simulink library "communications_lib"  (Simulink 8.1)
settings: Solver=ode45  StartTime=0.0  StopTime=10.0  RelTol=1e-3
values from neighbouring files (symbols this model uses):
  Ts = 100E-6    (= 0.0001)    [BANSHEE_init.m]    (also in Ghost_init.m)
libraries: goose_lib x6, rtlab x4, power_quality_lib x4, rtio_generic_modbus x2, DMS_slave_lib x2, LoadProfiles_lib x2, NREL_UDP_lib x2
(part 1 of 2)
settings Model: Creator=re25624  LastModifiedBy=hptb1

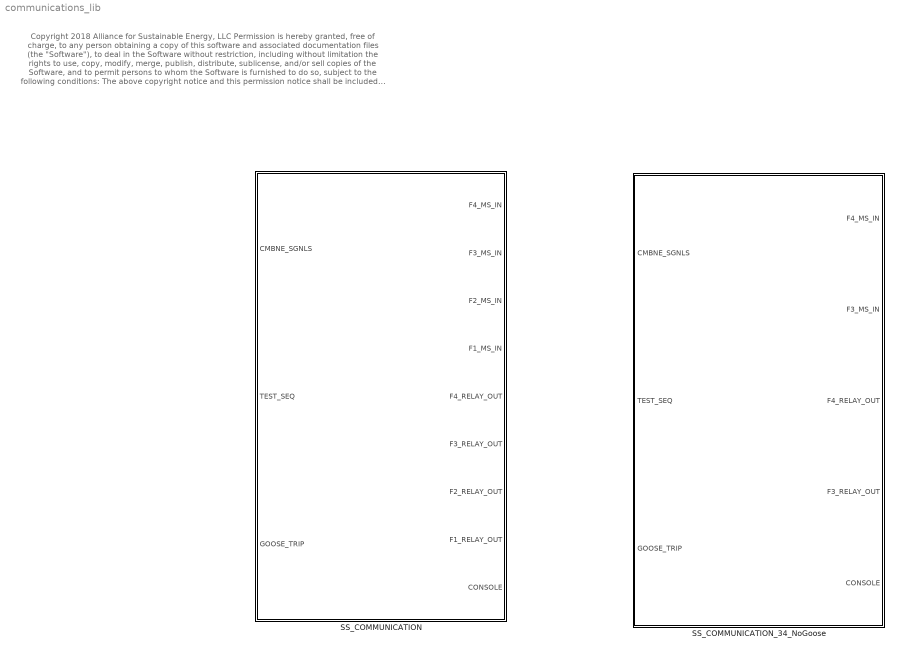
== system communications_lib ==
  note: Copyright 2018 Alliance for Sustainable Energy, LLC
      |
      | Permission is hereby granted, free of charge, to any person obtaining a copy of this software
      | and associated documentation files (the "Software"), to deal in the Software without restriction,
      | including without limitation the rights to use, copy, modify, merge, publish, distribute, sublicense,
      | and/or sell copies of the Software, and to permit persons to whom the Software is furnished to do so,
      | subject to the following conditions:
      |
      | The above copyright notice and this permission notice shall be included in all copies or substantial portions of the Software.
      |
      | THE SOFTWARE IS PROVIDED "AS IS", WITHOUT WARRANTY OF ANY KIND, EXPRESS OR IMPLIED, INCLUDING
      | BUT NOT LIMITED TO THE WARRANTIES OF MERCHANTABILITY, FITNESS FOR A PARTICULAR PURPOSE AND
      | NONINFRINGEMENT. IN NO EVENT SHALL THE AUTHORS, THE COPYRIGHT HOLDERS, THE UNITED STATES,
      | THE UNITED STATES DEPARTMENT OF ENERGY, OR ANY OF THEIR EMPLOYEES BE LIABLE FOR ANY CLAIM,
      | DAMAGES OR OTHER LIABILITY, WHETHER IN AN ACTION OF CONTRACT, TORT OR OTHERWISE, ARISING FROM,
      | OUT OF OR IN CONNECTION WITH THE SOFTWARE OR THE USE OR OTHER DEALINGS IN THE SOFTWARE.
  SS_COMMUNICATION : Subsystem
  SS_COMMUNICATION_34_NoGoose : Subsystem

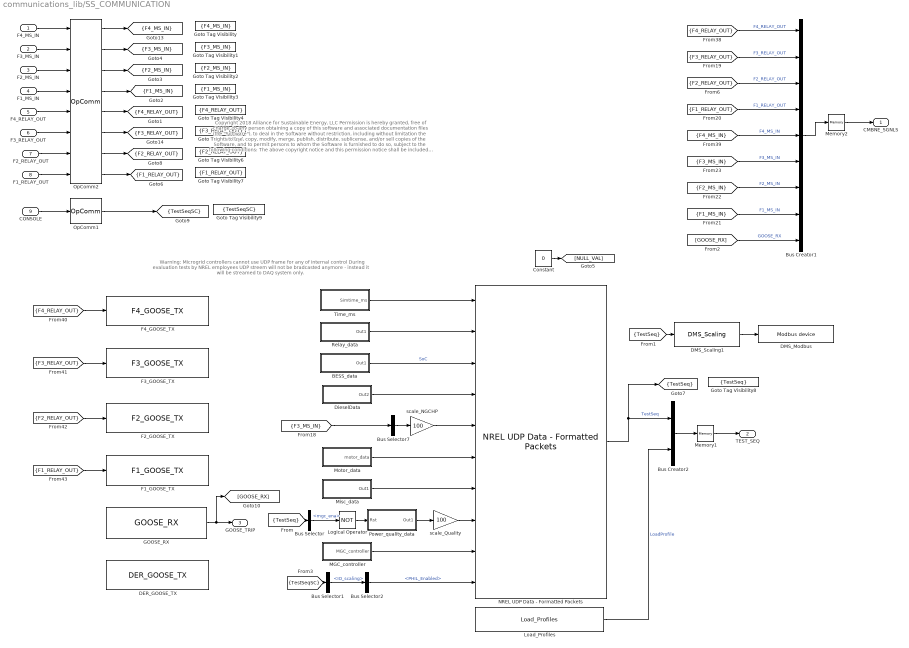
== system communications_lib/SS_COMMUNICATION ==
  note: Copyright 2018 Alliance for Sustainable Energy, LLC
      |
      | Permission is hereby granted, free of charge, to any person obtaining a copy of this software
      | and associated documentation files (the "Software"), to deal in the Software without restriction,
      | including without limitation the rights to use, copy, modify, merge, publish, distribute, sublicense,
      | and/or sell copies of the Software, and to permit persons to whom the Software is furnished to do so,
      | subject to the following conditions:
      |
      | The above copyright notice and this permission notice shall be included in all copies or substantial portions of the Software.
      |
      | THE SOFTWARE IS PROVIDED "AS IS", WITHOUT WARRANTY OF ANY KIND, EXPRESS OR IMPLIED, INCLUDING
      | BUT NOT LIMITED TO THE WARRANTIES OF MERCHANTABILITY, FITNESS FOR A PARTICULAR PURPOSE AND
      | NONINFRINGEMENT. IN NO EVENT SHALL THE AUTHORS, THE COPYRIGHT HOLDERS, THE UNITED STATES,
      | THE UNITED STATES DEPARTMENT OF ENERGY, OR ANY OF THEIR EMPLOYEES BE LIABLE FOR ANY CLAIM,
      | DAMAGES OR OTHER LIABILITY, WHETHER IN AN ACTION OF CONTRACT, TORT OR OTHERWISE, ARISING FROM,
      | OUT OF OR IN CONNECTION WITH THE SOFTWARE OR THE USE OR OTHER DEALINGS IN THE SOFTWARE.
  note: Warning: Microgrid controllers cannot use UDP frame for any of internal control
      | During evaluation tests by NREL employees UDP streem will not be bradcasted anymore - instead it will
      | be streamed to DAQ system only.
  F4_MS_IN : Inport
  F3_MS_IN : Inport  Port=2
  F2_MS_IN : Inport  Port=3
  F1_MS_IN : Inport  Port=4
  F4_RELAY_OUT : Inport  Port=5
  F3_RELAY_OUT : Inport  Port=6
  F2_RELAY_OUT : Inport  Port=7
  F1_RELAY_OUT : Inport  Port=8
  CONSOLE : Inport  Port=9
  BESS_data : Subsystem
  Bus Creator1 : BusCreator  Inputs=9
  Bus Creator2 : BusCreator  Inputs=2
  Bus Selector : BusSelector  OutputSignals=misc.mgc_ena
  Bus Selector1 : BusSelector  OutputSignals=IO_scaling
  Bus Selector2 : BusSelector  OutputSignals=PHIL_Enabled
  Bus Selector7 : BusSelector  OutputSignals=NG_CHP_DATA.cb.relay_out.m.Vpu,NG_CHP_DATA.CHPData.TempActual,NG_CHP_DATA.CHPData.Thermal data.Heat_Recovered_MBtu_hr,NG_CHP_DATA.CHPData.Thermal data.Nm3_per_hour_NG_fuel_usage,NG_CHP_DATA.CHPData.Thermal data.CO2_lbm_hr,NG_CHP_DATA.CHPData.HeatFromBoiler MBtu/hr,NG_CHP_DATA.CHPData.CHPHeatContribution MBtu/hr,NG_CHP_DATA.CHPData.Boiler_Nm^3/hr ,NG_CHP_DATA.CHPData.Boiler lbm/hr CO2  OutputAsBus=on
  Constant : Constant  Value=0
  DER_GOOSE_TX : goose_lib/DER_GOOSE_TX
  DMS_Modbus : rtio_generic_modbus/Modbus device  conf_name=DMS_cfg.opal  conf_name_mask=DMS_cfg.xls  sample_time=Ts
  DMS_Scaling1 : DMS_slave_lib/DMS_Scaling
  DieselData : Subsystem
  F1_GOOSE_TX : goose_lib/F1_GOOSE_TX
  F2_GOOSE_TX : goose_lib/F2_GOOSE_TX
  F3_GOOSE_TX : goose_lib/F3_GOOSE_TX
  F4_GOOSE_TX : goose_lib/F4_GOOSE_TX
  "GOOSE_RX " : goose_lib/GOOSE_RX 
  Goto Tag Visibility : GotoTagVisibility  GotoTag=F4_MS_IN
  Goto Tag Visibility1 : GotoTagVisibility  GotoTag=F3_MS_IN
  Goto Tag Visibility2 : GotoTagVisibility  GotoTag=F2_MS_IN
  Goto Tag Visibility3 : GotoTagVisibility  GotoTag=F1_MS_IN
  Goto Tag Visibility4 : GotoTagVisibility  GotoTag=F4_RELAY_OUT
  Goto Tag Visibility5 : GotoTagVisibility  GotoTag=F3_RELAY_OUT
  Goto Tag Visibility6 : GotoTagVisibility  GotoTag=F2_RELAY_OUT
  Goto Tag Visibility7 : GotoTagVisibility  GotoTag=F1_RELAY_OUT
  Goto Tag Visibility8 : GotoTagVisibility  GotoTag=TestSeq
  Goto Tag Visibility9 : GotoTagVisibility  GotoTag=TestSeqSC
  Load_Profiles : LoadProfiles_lib/Load_Profiles
  Logical Operator : Logic  Operator=NOT  AllPortsSameDT=off  OutDataTypeStr=boolean
  MGC_controller : Subsystem
  Memory1 : Memory
  Memory2 : Memory
  Misc_data : Subsystem
  Motor_data : Subsystem
  NREL UDP Data - Formatted Packets : NREL_UDP_lib/NREL UDP Data - Formatted Packets  ProfileID=6  NumOfRelays=[59, [1, 1, 1000, 100]]  NumOfBatteries=2  NumOfDieselGensets=[2, [100, 100]]  NumOfNGCHPGensets=[1, [100, 100, 100, 100, 100, 100, 100, 100, 100]]  NumOfMotors=2  NumOfQuality=[23 10 10]  NumOfMiscellaneousDataScales=2  NumOfMiscellaneousDataSignalsScales=[[50, 1], [8, 1]]
  OpComm1 : rtlab/OpComm  nbport=1  groupe_acq=1  subsys_rate=0  st=0  Synchronization=on  Interpolation=on  Threshold=1.0  Missed_Data=off  Sim_Time=off  Samples=off  dynSigOut=off  from_console=1  warning_done=off  writeOpCommFile=off  Offset=off
  OpComm2 : rtlab/OpComm  nbport=8  groupe_acq=1  subsys_rate=0  st=0  Synchronization=on  Interpolation=on  Threshold=1.0  Missed_Data=off  Sim_Time=off  Samples=off  dynSigOut=off  from_console=0  warning_done=off  writeOpCommFile=off  Offset=off
  Power_quality_data : Subsystem
  Relay_data : Subsystem
  Time_ms : Subsystem
  scale_NGCHP : Gain  Gain=100
  scale_Quality : Gain  Gain=100
  CMBNE_SGNLS : Outport
  TEST_SEQ : Outport  Port=2
  GOOSE_TRIP : Outport  Port=3
  tag scope: F1_MS_IN=scoped, F1_RELAY_OUT=scoped, F2_MS_IN=scoped, F2_RELAY_OUT=scoped, F3_MS_IN=scoped, F3_RELAY_OUT=scoped, F4_MS_IN=scoped, F4_RELAY_OUT=scoped, TestSeq=scoped, TestSeqSC=scoped
  wires:
  Bus Selector2/1 -> NREL UDP Data - Formatted Packets/10  "<PHIL_Enabled>"
  Bus Selector1/1 -> Bus Selector2/1  "<IO_scaling>"
  [TestSeqSC] -> Bus Selector1/1
  [GOOSE_RX] -> Bus Creator1/9  "GOOSE_RX"
  MGC_controller/1(MGC_controller) -> NREL UDP Data - Formatted Packets/9
  DMS_Scaling1/1 -> DMS_Modbus/1
  [TestSeq] -> DMS_Scaling1/1
  scale_Quality/1 -> NREL UDP Data - Formatted Packets/8
  Logical Operator/1 -> Power_quality_data/1(Rst)
  Bus Selector/1 -> Logical Operator/1  "<mgc_ena>"
  [TestSeq] -> Bus Selector/1
  Power_quality_data/1(Out1) -> scale_Quality/1
  DieselData/1(Out2) -> NREL UDP Data - Formatted Packets/4
  BESS_data/1(Out1) -> NREL UDP Data - Formatted Packets/3  "SoC"
  OpComm1/1 -> [TestSeqSC]
  CONSOLE/1 -> OpComm1/1
  Bus Creator2/1 -> Memory1/1
  NREL UDP Data - Formatted Packets/1 -> Bus Creator2/1, [TestSeq]  "TestSeq"
  Motor_data/1(motor_data) -> NREL UDP Data - Formatted Packets/6
  Misc_data/1(Out1) -> NREL UDP Data - Formatted Packets/7
  Relay_data/1(Out1) -> NREL UDP Data - Formatted Packets/2
  "GOOSE_RX "/1 -> GOOSE_TRIP/1, [GOOSE_RX]
  [F1_RELAY_OUT] -> F1_GOOSE_TX/1
  [F2_RELAY_OUT] -> F2_GOOSE_TX/1
  [F3_RELAY_OUT] -> F3_GOOSE_TX/1
  [F4_RELAY_OUT] -> F4_GOOSE_TX/1
  [F4_MS_IN] -> Bus Creator1/5  "F4_MS_IN"
  [F4_RELAY_OUT] -> Bus Creator1/1  "F4_RELAY_OUT"
  OpComm2/8 -> [F1_RELAY_OUT]
  OpComm2/7 -> [F2_RELAY_OUT]
  OpComm2/6 -> [F3_RELAY_OUT]
  OpComm2/5 -> [F4_RELAY_OUT]
  OpComm2/4 -> [F1_MS_IN]
  OpComm2/3 -> [F2_MS_IN]
  OpComm2/2 -> [F3_MS_IN]
  OpComm2/1 -> [F4_MS_IN]
  F3_RELAY_OUT/1 -> OpComm2/6
  F4_RELAY_OUT/1 -> OpComm2/5
  F4_MS_IN/1 -> OpComm2/1
  Time_ms/1(Simtime_ms) -> NREL UDP Data - Formatted Packets/1
  [F2_MS_IN] -> Bus Creator1/7  "F2_MS_IN"
  [F3_MS_IN] -> Bus Creator1/6  "F3_MS_IN"
  [F3_RELAY_OUT] -> Bus Creator1/2  "F3_RELAY_OUT"
  [F1_RELAY_OUT] -> Bus Creator1/4  "F1_RELAY_OUT"
  [F2_RELAY_OUT] -> Bus Creator1/3  "F2_RELAY_OUT"
  [F1_MS_IN] -> Bus Creator1/8  "F1_MS_IN"
  Bus Creator1/1 -> Memory2/1
  Memory2/1 -> CMBNE_SGNLS/1
  scale_NGCHP/1 -> NREL UDP Data - Formatted Packets/5
  Bus Selector7/1 -> scale_NGCHP/1
  [F3_MS_IN] -> Bus Selector7/1
  Constant/1 -> [NULL_VAL]
  F1_MS_IN/1 -> OpComm2/4
  F2_MS_IN/1 -> OpComm2/3
  F1_RELAY_OUT/1 -> OpComm2/8
  F2_RELAY_OUT/1 -> OpComm2/7
  Memory1/1 -> TEST_SEQ/1
  F3_MS_IN/1 -> OpComm2/2
  Load_Profiles/1 -> Bus Creator2/2  "LoadProfile"

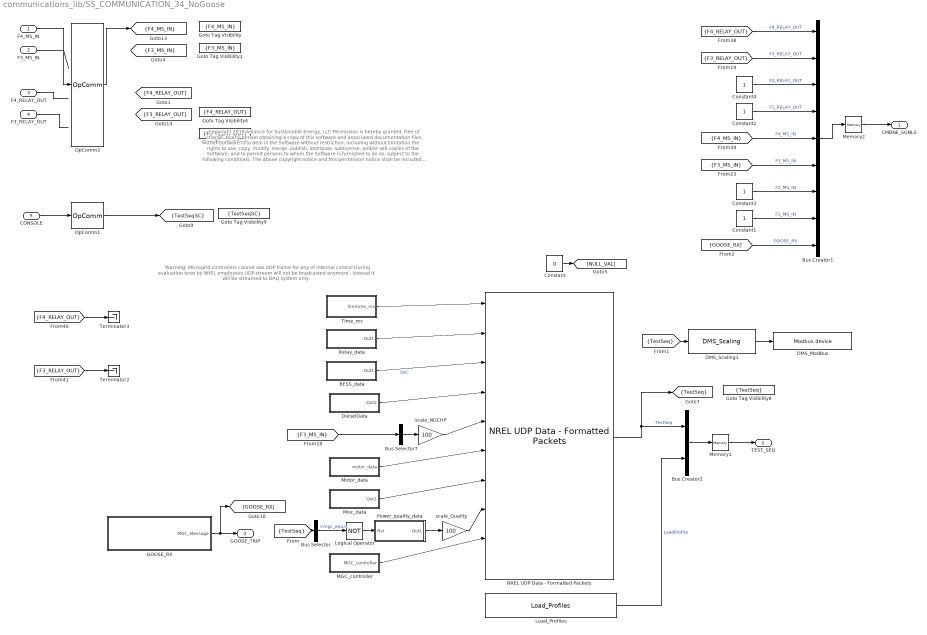
== system communications_lib/SS_COMMUNICATION_34_NoGoose ==
  note: Warning: Microgrid controllers cannot use UDP frame for any of internal control
      | During evaluation tests by NREL employees UDP streem will not be bradcasted anymore - instead it will
      | be streamed to DAQ system only.
  note: Copyright 2018 Alliance for Sustainable Energy, LLC
      |
      | Permission is hereby granted, free of charge, to any person obtaining a copy of this software
      | and associated documentation files (the "Software"), to deal in the Software without restriction,
      | including without limitation the rights to use, copy, modify, merge, publish, distribute, sublicense,
      | and/or sell copies of the Software, and to permit persons to whom the Software is furnished to do so,
      | subject to the following conditions:
      |
      | The above copyright notice and this permission notice shall be included in all copies or substantial portions of the Software.
      |
      | THE SOFTWARE IS PROVIDED "AS IS", WITHOUT WARRANTY OF ANY KIND, EXPRESS OR IMPLIED, INCLUDING
      | BUT NOT LIMITED TO THE WARRANTIES OF MERCHANTABILITY, FITNESS FOR A PARTICULAR PURPOSE AND
      | NONINFRINGEMENT. IN NO EVENT SHALL THE AUTHORS, THE COPYRIGHT HOLDERS, THE UNITED STATES,
      | THE UNITED STATES DEPARTMENT OF ENERGY, OR ANY OF THEIR EMPLOYEES BE LIABLE FOR ANY CLAIM,
      | DAMAGES OR OTHER LIABILITY, WHETHER IN AN ACTION OF CONTRACT, TORT OR OTHERWISE, ARISING FROM,
      | OUT OF OR IN CONNECTION WITH THE SOFTWARE OR THE USE OR OTHER DEALINGS IN THE SOFTWARE.
  F4_MS_IN : Inport
  F3_MS_IN : Inport  Port=2
  F4_RELAY_OUT : Inport  Port=3
  F3_RELAY_OUT : Inport  Port=4
  CONSOLE : Inport  Port=5
  BESS_data : Subsystem
  Bus Creator1 : BusCreator  Inputs=9
  Bus Creator2 : BusCreator  Inputs=2
  Bus Selector : BusSelector  OutputSignals=misc.mgc_ena
  Bus Selector7 : BusSelector  OutputSignals=NG_CHP_DATA.cb.relay_out.m.Vpu,NG_CHP_DATA.CHPData.TempActual,NG_CHP_DATA.CHPData.Thermal data.Heat_Recovered_MBtu_hr,NG_CHP_DATA.CHPData.Thermal data.Nm3_per_hour_NG_fuel_usage,NG_CHP_DATA.CHPData.Thermal data.CO2_lbm_hr,NG_CHP_DATA.CHPData.HeatFromBoiler MBtu/hr,NG_CHP_DATA.CHPData.CHPHeatContribution MBtu/hr,NG_CHP_DATA.CHPData.Boiler_Nm^3/hr ,NG_CHP_DATA.CHPData.Boiler lbm/hr CO2  OutputAsBus=on
  Constant : Constant  Value=0
  Constant{1..4} (4 alike) : Constant
  DMS_Modbus : rtio_generic_modbus/Modbus device  conf_name=DMS_cfg.opal  conf_name_mask=DMS_cfg.xls  sample_time=Ts
  DMS_Scaling1 : DMS_slave_lib/DMS_Scaling
  DieselData : Subsystem
  "GOOSE_RX " : Subsystem
  Goto Tag Visibility : GotoTagVisibility  GotoTag=F4_MS_IN
  Goto Tag Visibility1 : GotoTagVisibility  GotoTag=F3_MS_IN
  Goto Tag Visibility4 : GotoTagVisibility  GotoTag=F4_RELAY_OUT
  Goto Tag Visibility5 : GotoTagVisibility  GotoTag=F3_RELAY_OUT
  Goto Tag Visibility8 : GotoTagVisibility  GotoTag=TestSeq
  Goto Tag Visibility9 : GotoTagVisibility  GotoTag=TestSeqSC
  Load_Profiles : LoadProfiles_lib/Load_Profiles
  Logical Operator : Logic  Operator=NOT  AllPortsSameDT=off  OutDataTypeStr=boolean
  MGC_controller : Subsystem
  Memory1 : Memory
  Memory2 : Memory
  Misc_data : Subsystem
  Motor_data : Subsystem
  NREL UDP Data - Formatted Packets : NREL_UDP_lib/NREL UDP Data - Formatted Packets  ProfileID=6  NumOfRelays=[59, [1, 1, 1000, 100]]  NumOfBatteries=2  NumOfDieselGensets=[2, [100, 100]]  NumOfNGCHPGensets=[1, [100, 100, 100, 100, 100, 100, 100, 100, 100]]  NumOfMotors=2  NumOfQuality=[23 10 10]  NumOfMiscellaneousDataScales=2  NumOfMiscellaneousDataSignalsScales=[[50, 1], [8, 1]]
  OpComm1 : rtlab/OpComm  nbport=1  groupe_acq=1  subsys_rate=0  st=0  Synchronization=on  Interpolation=on  Threshold=1.0  Missed_Data=off  Sim_Time=off  Samples=off  dynSigOut=off  from_console=1  warning_done=off  writeOpCommFile=off  Offset=off
  OpComm2 : rtlab/OpComm  nbport=4  groupe_acq=1  subsys_rate=0  st=0  Synchronization=on  Interpolation=on  Threshold=1.0  Missed_Data=off  Sim_Time=off  Samples=off  dynSigOut=off  from_console=0  warning_done=off  writeOpCommFile=off  Offset=off
  Power_quality_data : Subsystem
  Relay_data : Subsystem
  Terminator2 : Terminator
  Terminator3 : Terminator
  Time_ms : Subsystem
  scale_NGCHP : Gain  Gain=100
  scale_Quality : Gain  Gain=100
  CMBNE_SGNLS : Outport
  TEST_SEQ : Outport  Port=2
  GOOSE_TRIP : Outport  Port=3
  tag scope: F3_MS_IN=scoped, F3_RELAY_OUT=scoped, F4_MS_IN=scoped, F4_RELAY_OUT=scoped, TestSeq=scoped, TestSeqSC=scoped
  wires:
  [GOOSE_RX] -> Bus Creator1/9  "GOOSE_RX"
  MGC_controller/1(MGC_controller) -> NREL UDP Data - Formatted Packets/9
  DMS_Scaling1/1 -> DMS_Modbus/1
  [TestSeq] -> DMS_Scaling1/1
  scale_Quality/1 -> NREL UDP Data - Formatted Packets/8
  Logical Operator/1 -> Power_quality_data/1(Rst)
  Bus Selector/1 -> Logical Operator/1  "<mgc_ena>"
  [TestSeq] -> Bus Selector/1
  Power_quality_data/1(Out1) -> scale_Quality/1
  DieselData/1(Out2) -> NREL UDP Data - Formatted Packets/4
  BESS_data/1(Out1) -> NREL UDP Data - Formatted Packets/3  "SoC"
  OpComm1/1 -> [TestSeqSC]
  CONSOLE/1 -> OpComm1/1
  Bus Creator2/1 -> Memory1/1
  NREL UDP Data - Formatted Packets/1 -> Bus Creator2/1, [TestSeq]  "TestSeq"
  Motor_data/1(motor_data) -> NREL UDP Data - Formatted Packets/6
  Misc_data/1(Out1) -> NREL UDP Data - Formatted Packets/7
  Relay_data/1(Out1) -> NREL UDP Data - Formatted Packets/2
  "GOOSE_RX "/1(MGC_Message) -> GOOSE_TRIP/1, [GOOSE_RX]
  [F3_RELAY_OUT] -> Terminator2/1
  [F4_RELAY_OUT] -> Terminator3/1
  [F4_MS_IN] -> Bus Creator1/5  "F4_MS_IN"
  [F4_RELAY_OUT] -> Bus Creator1/1  "F4_RELAY_OUT"
  ? -> [F3_RELAY_OUT]
  ? -> [F4_RELAY_OUT]
  ? -> [F3_MS_IN]
  OpComm2/1 -> [F4_MS_IN]
  F3_RELAY_OUT/1 -> ?
  F4_RELAY_OUT/1 -> ?
  F4_MS_IN/1 -> OpComm2/1
  Time_ms/1(Simtime_ms) -> NREL UDP Data - Formatted Packets/1
  Constant3/1 -> Bus Creator1/7  "F2_MS_IN"
  [F3_MS_IN] -> Bus Creator1/6  "F3_MS_IN"
  [F3_RELAY_OUT] -> Bus Creator1/2  "F3_RELAY_OUT"
  Constant2/1 -> Bus Creator1/4  "F1_RELAY_OUT"
  Constant4/1 -> Bus Creator1/3  "F2_RELAY_OUT"
  Constant1/1 -> Bus Creator1/8  "F1_MS_IN"
  Bus Creator1/1 -> Memory2/1
  Memory2/1 -> CMBNE_SGNLS/1
  scale_NGCHP/1 -> NREL UDP Data - Formatted Packets/5
  Bus Selector7/1 -> scale_NGCHP/1
  [F3_MS_IN] -> Bus Selector7/1
  Constant/1 -> [NULL_VAL]
  Memory1/1 -> TEST_SEQ/1
  F3_MS_IN/1 -> ?
  Load_Profiles/1 -> Bus Creator2/2  "LoadProfile"

== system communications_lib/SS_COMMUNICATION/BESS_data ==
  note: 0 .... 10000
      | 0 ... 100%
  Bus Selector1 : BusSelector  OutputSignals=Battery.SoC
  Bus Selector2 : BusSelector  OutputSignals=Battery.SoC
  Bus Selector3 : BusSelector  OutputSignals=ESS_DATA
  Bus Selector9 : BusSelector  OutputSignals=ESS_DATA
  Mux : Mux  Inputs=2
  Scale_SoC : Gain  Gain=100
  Out1 : Outport
  wires:
  [F2_MS_IN] -> Bus Selector3/1
  Bus Selector3/1 -> Bus Selector2/1  "<ESS_DATA>"
  Bus Selector2/1 -> Mux/1  "<SoC>"
  Scale_SoC/1 -> Out1/1
  [F4_MS_IN] -> Bus Selector9/1
  Bus Selector9/1 -> Bus Selector1/1  "<ESS_DATA>"
  Bus Selector1/1 -> Mux/2  "<SoC>"
  Mux/1 -> Scale_SoC/1

== system communications_lib/SS_COMMUNICATION/DieselData ==
  Bus Selector : BusSelector  OutputSignals=GEN3_DATA.gen.gal_per_hr,GEN3_DATA.cb.relay_out.m.Vpu
  Bus Selector1 : BusSelector  OutputSignals=DIESEL_DATA.gen.gal_per_hr,DIESEL_DATA.cb.relay_out.m.Vpu
  Mux : Mux
  scale_diesel3 : Gain  Gain=100
  Out2 : Outport
  wires:
  Bus Selector1/2 -> Mux/3  "<Vpu>"
  scale_diesel3/1 -> Out2/1
  [F1_MS_IN] -> Bus Selector1/1
  [F4_MS_IN] -> Bus Selector/1
  Bus Selector/1 -> Mux/2  "<gal_per_hr>"
  Bus Selector1/1 -> Mux/1  "<gal_per_hr>"
  Mux/1 -> scale_diesel3/1
  Bus Selector/2 -> Mux/4  "<Vpu>"

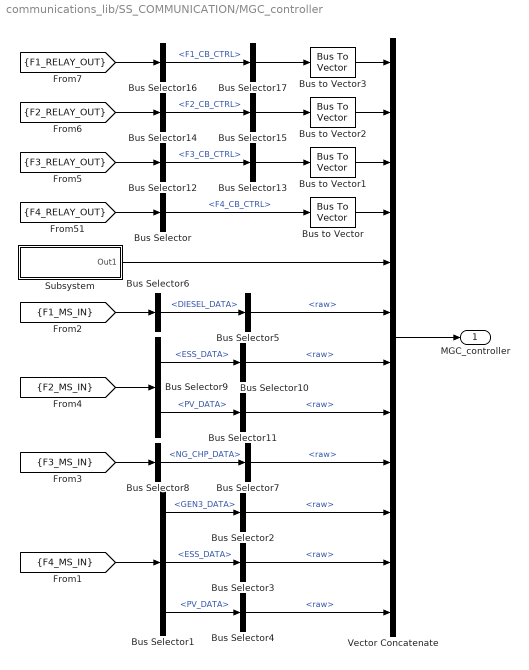
== system communications_lib/SS_COMMUNICATION/MGC_controller ==
  Bus Selector : BusSelector  OutputSignals=F4_CB_CTRL
  Bus Selector1 : BusSelector  OutputSignals=GEN3_DATA,ESS_DATA,PV_DATA
  Bus Selector{3..4,10..11} (4 alike) : BusSelector  OutputSignals=raw
  Bus Selector12 : BusSelector  OutputSignals=F3_CB_CTRL
  Bus Selector13 : BusSelector  OutputSignals=signal1,signal2,signal3,signal4,signal5,signal6,signal7,signal8,signal9,signal10  OutputAsBus=on
  Bus Selector14 : BusSelector  OutputSignals=F2_CB_CTRL
  Bus Selector15 : BusSelector  OutputSignals=signal1,signal2,signal3,signal4,signal5,signal6,signal7,signal8,signal9,signal10,signal11,signal12,signal13,signal14,signal15,signal16,signal17,signal18,signal19  OutputAsBus=on
  Bus Selector16 : BusSelector  OutputSignals=F1_CB_CTRL
  Bus Selector17 : BusSelector  OutputSignals=signal1,signal2,signal3,signal4,signal5,signal6,signal7,signal8,signal9,signal10,signal11,signal12,signal13,signal14  OutputAsBus=on
  Bus Selector2 : BusSelector  OutputSignals=ctrl.raw
  Bus Selector5 : BusSelector  OutputSignals=ctrl.raw
  Bus Selector6 : BusSelector  OutputSignals=DIESEL_DATA
  Bus Selector7 : BusSelector  OutputSignals=ctrl.raw
  Bus Selector8 : BusSelector  OutputSignals=NG_CHP_DATA
  Bus Selector9 : BusSelector  OutputSignals=ESS_DATA,PV_DATA
  Bus to Vector{,1..3} (4 alike) : BusToVector
  Subsystem : Subsystem
      mask Display: disp('PCC control');
  Vector Concatenate : Concatenate  NumInputs=12
  MGC_controller : Outport
  wires:
  Bus Selector17/1 -> Bus to Vector3/1
  Bus Selector16/1 -> Bus Selector17/1  "<F1_CB_CTRL>"
  [F1_RELAY_OUT] -> Bus Selector16/1
  Bus to Vector3/1 -> Vector Concatenate/1
  Bus Selector15/1 -> Bus to Vector2/1
  Bus Selector14/1 -> Bus Selector15/1  "<F2_CB_CTRL>"
  [F2_RELAY_OUT] -> Bus Selector14/1
  Bus to Vector2/1 -> Vector Concatenate/2
  Bus Selector13/1 -> Bus to Vector1/1
  Bus Selector12/1 -> Bus Selector13/1  "<F3_CB_CTRL>"
  [F3_RELAY_OUT] -> Bus Selector12/1
  Bus to Vector/1 -> Vector Concatenate/4
  Bus Selector9/2 -> Bus Selector11/1  "<PV_DATA>"
  Bus Selector9/1 -> Bus Selector10/1  "<ESS_DATA>"
  Bus Selector11/1 -> Vector Concatenate/8  "<raw>"
  Bus Selector10/1 -> Vector Concatenate/7  "<raw>"
  [F2_MS_IN] -> Bus Selector9/1
  Bus Selector4/1 -> Vector Concatenate/12  "<raw>"
  Bus Selector8/1 -> Bus Selector7/1  "<NG_CHP_DATA>"
  [F3_MS_IN] -> Bus Selector8/1
  Bus Selector7/1 -> Vector Concatenate/9  "<raw>"
  Bus Selector6/1 -> Bus Selector5/1  "<DIESEL_DATA>"
  [F1_MS_IN] -> Bus Selector6/1
  Vector Concatenate/1 -> MGC_controller/1
  Subsystem/1(Out1) -> Vector Concatenate/5
  Bus to Vector1/1 -> Vector Concatenate/3
  Bus Selector/1 -> Bus to Vector/1  "<F4_CB_CTRL>"
  [F4_RELAY_OUT] -> Bus Selector/1
  [F4_MS_IN] -> Bus Selector1/1
  Bus Selector1/1 -> Bus Selector2/1  "<GEN3_DATA>"
  Bus Selector1/2 -> Bus Selector3/1  "<ESS_DATA>"
  Bus Selector1/3 -> Bus Selector4/1  "<PV_DATA>"
  Bus Selector3/1 -> Vector Concatenate/11  "<raw>"
  Bus Selector2/1 -> Vector Concatenate/10  "<raw>"
  Bus Selector5/1 -> Vector Concatenate/6  "<raw>"

== system communications_lib/SS_COMMUNICATION/Misc_data ==
  note: Data ordered as:
      | I-P-C
      | kW-VRMSLL
  Bus Creator : BusCreator
  Constant : Constant  Value=zeros(1,9)
  Mux8 : Mux  Inputs=2
  Mux9 : Mux  Inputs=2
  Subsystem : Subsystem
  Subsystem1 : Subsystem
  scale_load : Gain
  Out1 : Outport
  wires:
  Subsystem1/1(Out1) -> Mux8/2
  Subsystem/1(Out1) -> Mux8/1
  [F4_MS_IN] -> Bus Creator/1  "F4"
  Mux9/1 -> Out1/1
  Constant/1 -> Mux9/2
  Mux8/1 -> scale_load/1
  Bus Creator/1 -> Subsystem/1(In1), Subsystem1/1(In1)
  [F1_MS_IN] -> Bus Creator/4  "F1"
  [F2_MS_IN] -> Bus Creator/3  "F2"
  [F3_MS_IN] -> Bus Creator/2  "F3"
  scale_load/1 -> Mux9/1

== system communications_lib/SS_COMMUNICATION/Motor_data ==
  note: kW
      | kVAR
      | VLL_RMS
      | RPM
  Bus Selector1 : BusSelector  OutputSignals=MOTOR_DATA
  Bus Selector2 : BusSelector  OutputSignals=kW,kVAr,VRMSLL,RPM  OutputAsBus=on
  Bus Selector3 : BusSelector  OutputSignals=MOTOR_DATA
  Bus Selector4 : BusSelector  OutputSignals=kW,kVAr,VRMSLL,RPM  OutputAsBus=on
  Bus to Vector : BusToVector
  Bus to Vector1 : BusToVector
  Mux5 : Mux  Inputs=2
  motor_data : Outport
  wires:
  Bus Selector4/1 -> Bus to Vector1/1
  Bus Selector3/1 -> Bus Selector4/1  "<MOTOR_DATA>"
  [F3_MS_IN] -> Bus Selector3/1
  Bus to Vector1/1 -> Mux5/2  "Motor2"
  Bus Selector2/1 -> Bus to Vector/1
  Bus Selector1/1 -> Bus Selector2/1  "<MOTOR_DATA>"
  [F1_MS_IN] -> Bus Selector1/1
  Bus to Vector/1 -> Mux5/1  "Motor1"
  Mux5/1 -> motor_data/1

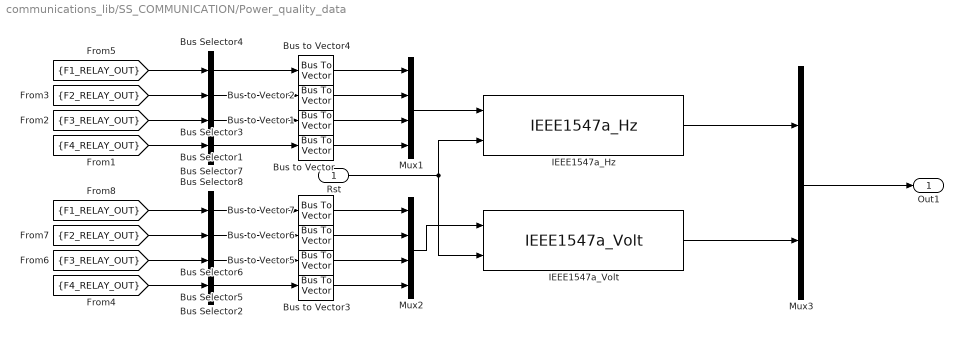
== system communications_lib/SS_COMMUNICATION/Power_quality_data ==
  Rst : Inport
  Bus Selector1 : BusSelector  OutputSignals=F3_CB_1.m.Hz,F3_CB_5.m.Hz,F3_CB_7.m.Hz,F3_CB_8.m.Hz,F3_CB_9.m.Hz  OutputAsBus=on
  Bus Selector2 : BusSelector  OutputSignals=F4_CB_1.m.Vpu,F4_CB_2.m.Vpu,F4_CB_5.m.Vpu  OutputAsBus=on
  Bus Selector3 : BusSelector  OutputSignals=F2_CB_1.m.Hz,F2_CB_6.m.Hz,F2_CB_8.m.Hz,F2_CB_9.m.Hz,F2_CB_12.m.Hz,F2_CB_14.m.Hz,F2_CB_16.m.Hz,F2_CB_17.m.Hz,F2_CB_19.m.Hz  OutputAsBus=on
  Bus Selector4 : BusSelector  OutputSignals=F1_CB_1.m.Hz,F1_CB_4.m.Hz,F1_CB_9.m.Hz,F1_CB_6.m.Hz,F1_CB_10.m.Hz,F1_CB_14.m.Hz  OutputAsBus=on
  Bus Selector5 : BusSelector  OutputSignals=F3_CB_1.m.Vpu,F3_CB_5.m.Vpu,F3_CB_7.m.Vpu,F3_CB_8.m.Vpu,F3_CB_9.m.Vpu  OutputAsBus=on
  Bus Selector6 : BusSelector  OutputSignals=F2_CB_1.m.Vpu,F2_CB_6.m.Vpu,F2_CB_8.m.Vpu,F2_CB_9.m.Vpu,F2_CB_12.m.Vpu,F2_CB_14.m.Vpu,F2_CB_16.m.Vpu,F2_CB_17.m.Vpu,F2_CB_19.m.Vpu  OutputAsBus=on
  Bus Selector7 : BusSelector  OutputSignals=F4_CB_1.m.Hz,F4_CB_2.m.Hz,F4_CB_5.m.Hz  OutputAsBus=on
  Bus Selector8 : BusSelector  OutputSignals=F1_CB_1.m.Vpu,F1_CB_4.m.Vpu,F1_CB_9.m.Vpu,F1_CB_6.m.Vpu,F1_CB_10.m.Vpu,F1_CB_14.m.Vpu  OutputAsBus=on
  Bus to Vector{,1..7} (8 alike) : BusToVector
  IEEE1547a_Hz : power_quality_lib/IEEE1547a_Hz
  IEEE1547a_Volt : power_quality_lib/IEEE1547a_Volt
  Mux1 : Mux
  Mux2 : Mux
  Mux3 : Mux  Inputs=2
  Out1 : Outport
  wires:
  Mux2/1 -> IEEE1547a_Volt/1
  Bus to Vector7/1 -> Mux2/1
  Bus Selector8/1 -> Bus to Vector7/1
  [F1_RELAY_OUT] -> Bus Selector8/1
  Bus to Vector6/1 -> Mux2/2
  Bus Selector6/1 -> Bus to Vector6/1
  [F2_RELAY_OUT] -> Bus Selector6/1
  Bus to Vector5/1 -> Mux2/3
  Bus Selector5/1 -> Bus to Vector5/1
  [F3_RELAY_OUT] -> Bus Selector5/1
  Mux1/1 -> IEEE1547a_Hz/1
  Bus to Vector1/1 -> Mux1/3
  Bus to Vector2/1 -> Mux1/2
  Bus to Vector4/1 -> Mux1/1
  Bus Selector1/1 -> Bus to Vector1/1
  Bus Selector3/1 -> Bus to Vector2/1
  Bus Selector4/1 -> Bus to Vector4/1
  [F3_RELAY_OUT] -> Bus Selector1/1
  [F2_RELAY_OUT] -> Bus Selector3/1
  [F1_RELAY_OUT] -> Bus Selector4/1
  Bus to Vector3/1 -> Mux2/4
  Bus Selector2/1 -> Bus to Vector3/1
  [F4_RELAY_OUT] -> Bus Selector7/1
  [F4_RELAY_OUT] -> Bus Selector2/1
  Bus to Vector/1 -> Mux1/4
  IEEE1547a_Hz/1 -> Mux3/1
  IEEE1547a_Volt/1 -> Mux3/2
  Mux3/1 -> Out1/1
  Bus Selector7/1 -> Bus to Vector/1
  Rst/1 -> IEEE1547a_Hz/2, IEEE1547a_Volt/2

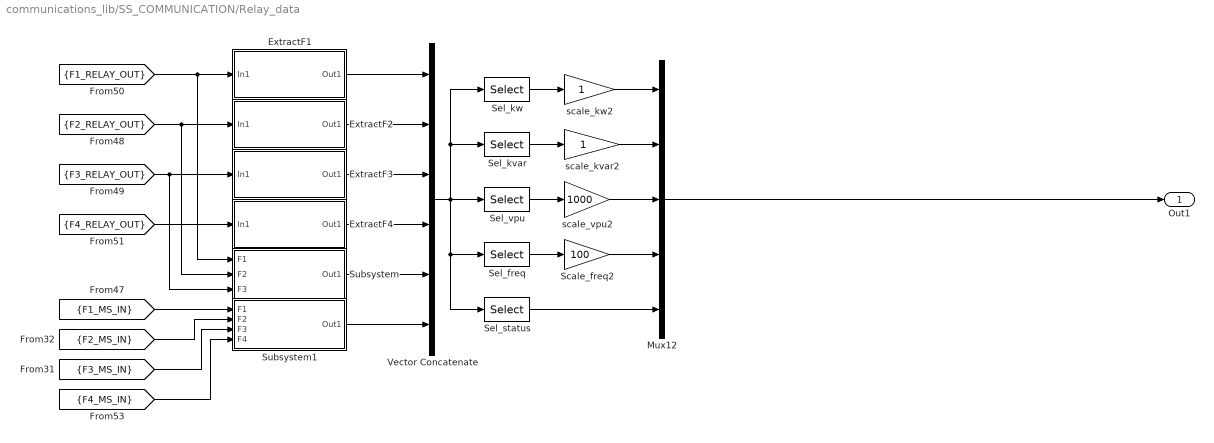
== system communications_lib/SS_COMMUNICATION/Relay_data ==
  ExtractF1 : Subsystem
      mask Display: disp('Generic F1 relays\nID = 01 .. 14')
  ExtractF2 : Subsystem
      mask Display: disp('Generic F2 relays\nID = 15 .. 33')
  ExtractF3 : Subsystem
      mask Display: disp('Generic F3 relays\nID = 34 .. 43')
  ExtractF4 : Subsystem
      mask Display: disp('Generic F4 relays\nID = 44 .. 49')
  Mux12 : Mux  Inputs=5
  Scale_freq2 : Gain  Gain=100
  Sel_freq : Selector  InputPortWidth=59*5  IndexOptions=Index vector (dialog)  Indices=[4:5:59*5]  OutputSizes=1
  Sel_kvar : Selector  InputPortWidth=59*5  IndexOptions=Index vector (dialog)  Indices=[2:5:59*5]  OutputSizes=1
  Sel_kw : Selector  InputPortWidth=59*5  IndexOptions=Index vector (dialog)  Indices=[1:5:59*5]  OutputSizes=1
  Sel_status : Selector  InputPortWidth=59*5  IndexOptions=Index vector (dialog)  Indices=[5:5:59*5]  OutputSizes=1
  Sel_vpu : Selector  InputPortWidth=59*5  IndexOptions=Index vector (dialog)  Indices=[3:5:59*5]  OutputSizes=1
  Subsystem : Subsystem
      mask Display: disp('Generic PCC relays\nID = 50 .. 52')
  Subsystem1 : Subsystem
      mask Display: disp('GEN1,ESS1,PV1\nGEN2,GEN3,ESS2,PV1\nID = 53 .. 59')
  Vector Concatenate : Concatenate  NumInputs=6
  scale_kvar2 : Gain
  scale_kw2 : Gain
  scale_vpu2 : Gain  Gain=1000
  Out1 : Outport
  wires:
  Vector Concatenate/1 -> Sel_kw/1, Sel_kvar/1, Sel_vpu/1, Sel_freq/1, Sel_status/1
  Sel_kvar/1 -> scale_kvar2/1
  Sel_vpu/1 -> scale_vpu2/1
  Sel_freq/1 -> Scale_freq2/1
  Sel_status/1 -> Mux12/5
  Sel_kw/1 -> scale_kw2/1
  scale_vpu2/1 -> Mux12/3
  Scale_freq2/1 -> Mux12/4
  scale_kvar2/1 -> Mux12/2
  scale_kw2/1 -> Mux12/1
  Mux12/1 -> Out1/1
  Subsystem1/1(Out1) -> Vector Concatenate/6
  [F1_MS_IN] -> Subsystem1/1(F1)
  [F2_MS_IN] -> Subsystem1/2(F2)
  [F3_MS_IN] -> Subsystem1/3(F3)
  [F4_MS_IN] -> Subsystem1/4(F4)
  Subsystem/1(Out1) -> Vector Concatenate/5
  ExtractF1/1(Out1) -> Vector Concatenate/1
  ExtractF2/1(Out1) -> Vector Concatenate/2
  ExtractF3/1(Out1) -> Vector Concatenate/3
  ExtractF4/1(Out1) -> Vector Concatenate/4
  [F4_RELAY_OUT] -> ExtractF4/1(In1)
  [F2_RELAY_OUT] -> ExtractF2/1(In1), Subsystem/2(F2)
  [F1_RELAY_OUT] -> ExtractF1/1(In1), Subsystem/1(F1)
  [F3_RELAY_OUT] -> ExtractF3/1(In1), Subsystem/3(F3)

== system communications_lib/SS_COMMUNICATION/Time_ms ==
  Constant4 : Constant  Value=Ts/1e-3
  Sum : Sum  Inputs=++|
  Unit Delay : UnitDelay  SampleTime=-1
  Simtime_ms : Outport
  wires:
  Sum/1 -> Simtime_ms/1, Unit Delay/1
  Constant4/1 -> Sum/2
  Unit Delay/1 -> Sum/1

== system communications_lib/SS_COMMUNICATION_34_NoGoose/BESS_data ==
  note: 0 .... 10000
      | 0 ... 100%
  Bus Selector1 : BusSelector  OutputSignals=Battery.SoC
  Bus Selector9 : BusSelector  OutputSignals=ESS_DATA
  Constant : Constant  Value=0
  Mux : Mux  Inputs=2
  Scale_SoC : Gain  Gain=100
  Out1 : Outport
  wires:
  Constant/1 -> Mux/1
  Scale_SoC/1 -> Out1/1
  [F4_MS_IN] -> Bus Selector9/1
  Bus Selector9/1 -> Bus Selector1/1  "<ESS_DATA>"
  Bus Selector1/1 -> Mux/2  "<SoC>"
  Mux/1 -> Scale_SoC/1

== system communications_lib/SS_COMMUNICATION_34_NoGoose/DieselData ==
  Bus Selector : BusSelector  OutputSignals=GEN3_DATA.gen.gal_per_hr,GEN3_DATA.cb.relay_out.m.Vpu
  Constant : Constant  Value=0
  Constant1 : Constant  Value=0
  Mux : Mux
  scale_diesel3 : Gain  Gain=100
  Out2 : Outport
  wires:
  Constant1/1 -> Mux/3
  scale_diesel3/1 -> Out2/1
  [F4_MS_IN] -> Bus Selector/1
  Bus Selector/1 -> Mux/2  "<gal_per_hr>"
  Constant/1 -> Mux/1
  Mux/1 -> scale_diesel3/1
  Bus Selector/2 -> Mux/4  "<Vpu>"

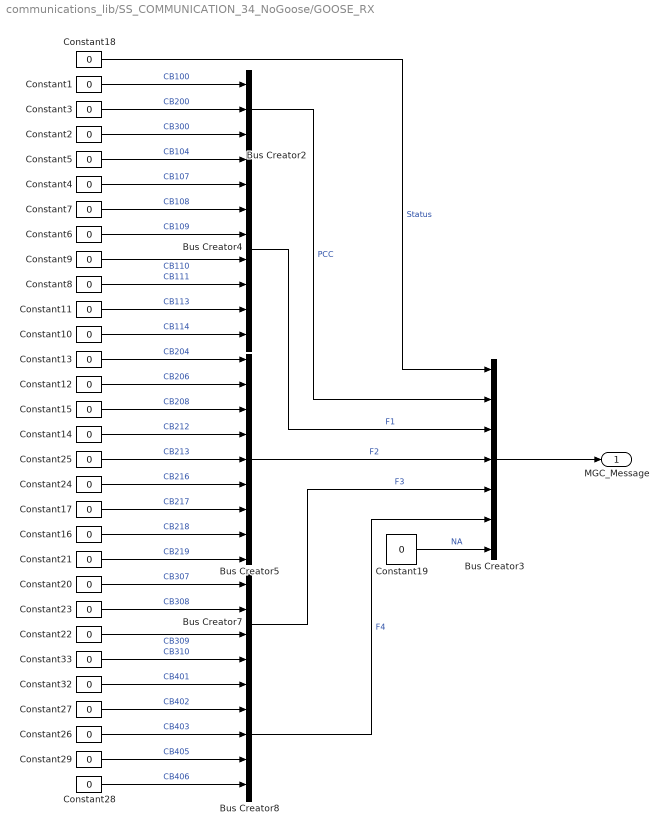
== system communications_lib/SS_COMMUNICATION_34_NoGoose/GOOSE_RX  ==
  Bus Creator2 : BusCreator  Inputs=3
  Bus Creator3 : BusCreator  Inputs=7
  Bus Creator4 : BusCreator  Inputs=8
  Bus Creator5 : BusCreator  Inputs=9
  Bus Creator7 : BusCreator
  Bus Creator8 : BusCreator  Inputs=5
  Constant{1..29,32..33} (31 alike) : Constant  Value=0
  MGC_Message : Outport
  wires:
  Constant32/1 -> Bus Creator8/1  "CB401"
  Constant27/1 -> Bus Creator8/2  "CB402"
  Constant29/1 -> Bus Creator8/4  "CB405"
  Constant19/1 -> Bus Creator3/7  "NA"
  Constant20/1 -> Bus Creator7/1  "CB307"
  Constant23/1 -> Bus Creator7/2  "CB308"
  Constant22/1 -> Bus Creator7/3  "CB309"
  Constant33/1 -> Bus Creator7/4  "CB310"
  Bus Creator7/1 -> Bus Creator3/5  "F3"
  Constant26/1 -> Bus Creator8/3  "CB403"
  Constant28/1 -> Bus Creator8/5  "CB406"
  Bus Creator8/1 -> Bus Creator3/6  "F4"
  Bus Creator5/1 -> Bus Creator3/4  "F2"
  Constant12/1 -> Bus Creator5/2  "CB206"
  Constant14/1 -> Bus Creator5/4  "CB212"
  Constant13/1 -> Bus Creator5/1  "CB204"
  Constant15/1 -> Bus Creator5/3  "CB208"
  Constant16/1 -> Bus Creator5/8  "CB218"
  Constant25/1 -> Bus Creator5/5  "CB213"
  Constant17/1 -> Bus Creator5/7  "CB217"
  Constant24/1 -> Bus Creator5/6  "CB216"
  Constant21/1 -> Bus Creator5/9  "CB219"
  Bus Creator4/1 -> Bus Creator3/3  "F1"
  Constant10/1 -> Bus Creator4/8  "CB114"
  Constant11/1 -> Bus Creator4/7  "CB113"
  Constant8/1 -> Bus Creator4/6  "CB111"
  Constant5/1 -> Bus Creator4/1  "CB104"
  Constant9/1 -> Bus Creator4/5  "CB110"
  Constant4/1 -> Bus Creator4/2  "CB107"
  Constant6/1 -> Bus Creator4/4  "CB109"
  Constant7/1 -> Bus Creator4/3  "CB108"
  Bus Creator2/1 -> Bus Creator3/2  "PCC"
  Constant2/1 -> Bus Creator2/3  "CB300"
  Constant3/1 -> Bus Creator2/2  "CB200"
  Constant1/1 -> Bus Creator2/1  "CB100"
  Bus Creator3/1 -> MGC_Message/1
  Constant18/1 -> Bus Creator3/1  "Status"

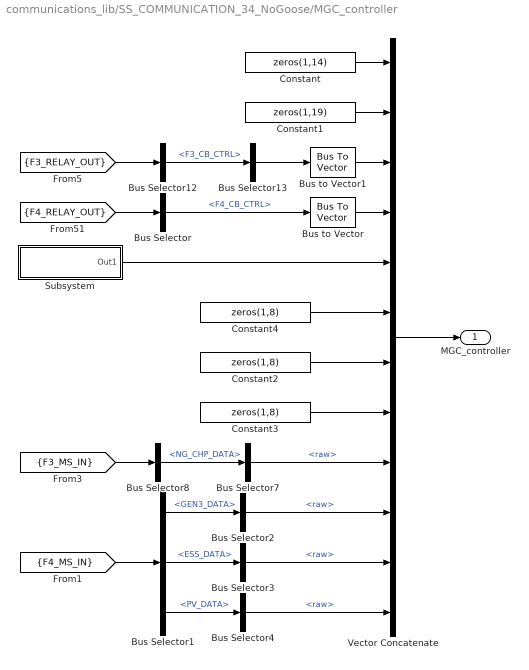
== system communications_lib/SS_COMMUNICATION_34_NoGoose/MGC_controller ==
  Bus Selector : BusSelector  OutputSignals=F4_CB_CTRL
  Bus Selector1 : BusSelector  OutputSignals=GEN3_DATA,ESS_DATA,PV_DATA
  Bus Selector12 : BusSelector  OutputSignals=F3_CB_CTRL
  Bus Selector13 : BusSelector  OutputSignals=signal1,signal2,signal3,signal4,signal5,signal6,signal7,signal8,signal9,signal10  OutputAsBus=on
  Bus Selector2 : BusSelector  OutputSignals=ctrl.raw
  Bus Selector3 : BusSelector  OutputSignals=raw
  Bus Selector4 : BusSelector  OutputSignals=raw
  Bus Selector7 : BusSelector  OutputSignals=ctrl.raw
  Bus Selector8 : BusSelector  OutputSignals=NG_CHP_DATA
  Bus to Vector : BusToVector
  Bus to Vector1 : BusToVector
  Constant : Constant  Value=zeros(1,14)
  Constant1 : Constant  Value=zeros(1,19)
  Constant2 : Constant  Value=zeros(1,8)
  Constant3 : Constant  Value=zeros(1,8)
  Constant4 : Constant  Value=zeros(1,8)
  Subsystem : Subsystem
      mask Display: disp('PCC control');
  Vector Concatenate : Concatenate  NumInputs=12
  MGC_controller : Outport
  wires:
  Constant3/1 -> Vector Concatenate/8
  Constant2/1 -> Vector Concatenate/7
  Constant4/1 -> Vector Concatenate/6
  Constant/1 -> Vector Concatenate/1
  Constant1/1 -> Vector Concatenate/2
  Bus Selector13/1 -> Bus to Vector1/1
  Bus Selector12/1 -> Bus Selector13/1  "<F3_CB_CTRL>"
  [F3_RELAY_OUT] -> Bus Selector12/1
  Bus to Vector/1 -> Vector Concatenate/4
  Bus Selector4/1 -> Vector Concatenate/12  "<raw>"
  Bus Selector8/1 -> Bus Selector7/1  "<NG_CHP_DATA>"
  [F3_MS_IN] -> Bus Selector8/1
  Bus Selector7/1 -> Vector Concatenate/9  "<raw>"
  Vector Concatenate/1 -> MGC_controller/1
  Subsystem/1(Out1) -> Vector Concatenate/5
  Bus to Vector1/1 -> Vector Concatenate/3
  Bus Selector/1 -> Bus to Vector/1  "<F4_CB_CTRL>"
  [F4_RELAY_OUT] -> Bus Selector/1
  [F4_MS_IN] -> Bus Selector1/1
  Bus Selector1/1 -> Bus Selector2/1  "<GEN3_DATA>"
  Bus Selector1/2 -> Bus Selector3/1  "<ESS_DATA>"
  Bus Selector1/3 -> Bus Selector4/1  "<PV_DATA>"
  Bus Selector3/1 -> Vector Concatenate/11  "<raw>"
  Bus Selector2/1 -> Vector Concatenate/10  "<raw>"

== system communications_lib/SS_COMMUNICATION_34_NoGoose/Misc_data ==
  note: Data ordered as:
      | I-P-C
      | kW-VRMSLL
  Bus Creator : BusCreator
  Constant : Constant  Value=zeros(1,9)
  Constant1 : Constant  Value=0
  Constant2 : Constant  Value=0
  Mux8 : Mux  Inputs=2
  Mux9 : Mux  Inputs=2
  Subsystem : Subsystem
  Subsystem1 : Subsystem
  scale_load : Gain
  Out1 : Outport
  wires:
  Subsystem1/1(Out1) -> Mux8/2
  Subsystem/1(Out1) -> Mux8/1
  [F4_MS_IN] -> Bus Creator/1  "F4"
  Mux9/1 -> Out1/1
  Constant/1 -> Mux9/2
  Mux8/1 -> scale_load/1
  Bus Creator/1 -> Subsystem/1(In1), Subsystem1/1(In1)
  Constant1/1 -> Bus Creator/4  "F1"
  Constant2/1 -> Bus Creator/3  "F2"
  [F3_MS_IN] -> Bus Creator/2  "F3"
  scale_load/1 -> Mux9/1

== system communications_lib/SS_COMMUNICATION_34_NoGoose/Motor_data ==
  note: kW
      | kVAR
      | VLL_RMS
      | RPM
  Bus Selector3 : BusSelector  OutputSignals=MOTOR_DATA
  Bus Selector4 : BusSelector  OutputSignals=kW,kVAr,VRMSLL,RPM  OutputAsBus=on
  Bus to Vector1 : BusToVector
  Constant : Constant  Value=zeros(4,1)
  Mux5 : Mux  Inputs=2
  motor_data : Outport
  wires:
  Bus Selector4/1 -> Bus to Vector1/1
  Bus Selector3/1 -> Bus Selector4/1  "<MOTOR_DATA>"
  [F3_MS_IN] -> Bus Selector3/1
  Bus to Vector1/1 -> Mux5/2  "Motor2"
  Constant/1 -> Mux5/1  "Motor1"
  Mux5/1 -> motor_data/1

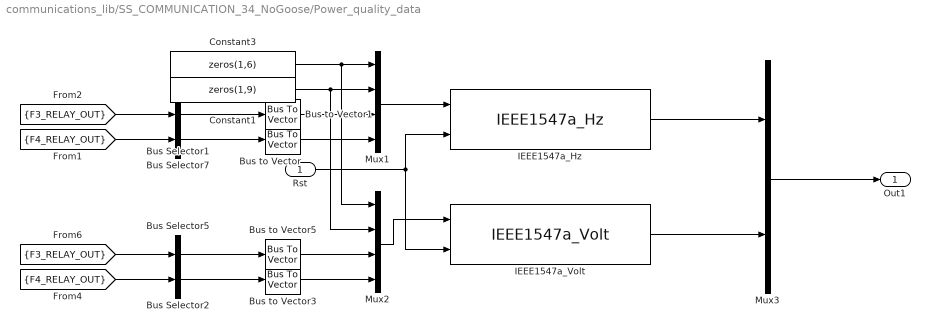
== system communications_lib/SS_COMMUNICATION_34_NoGoose/Power_quality_data ==
  Rst : Inport
  Bus Selector1 : BusSelector  OutputSignals=F3_CB_1.m.Hz,F3_CB_5.m.Hz,F3_CB_7.m.Hz,F3_CB_8.m.Hz,F3_CB_9.m.Hz  OutputAsBus=on
  Bus Selector2 : BusSelector  OutputSignals=F4_CB_1.m.Vpu,F4_CB_2.m.Vpu,F4_CB_5.m.Vpu  OutputAsBus=on
  Bus Selector5 : BusSelector  OutputSignals=F3_CB_1.m.Vpu,F3_CB_5.m.Vpu,F3_CB_7.m.Vpu,F3_CB_8.m.Vpu,F3_CB_9.m.Vpu  OutputAsBus=on
  Bus Selector7 : BusSelector  OutputSignals=F4_CB_1.m.Hz,F4_CB_2.m.Hz,F4_CB_5.m.Hz  OutputAsBus=on
  Bus to Vector{,1,3,5} (4 alike) : BusToVector
  Constant1 : Constant  Value=zeros(1,9)
  Constant3 : Constant  Value=zeros(1,6)
  IEEE1547a_Hz : power_quality_lib/IEEE1547a_Hz
  IEEE1547a_Volt : power_quality_lib/IEEE1547a_Volt
  Mux1 : Mux
  Mux2 : Mux
  Mux3 : Mux  Inputs=2
  Out1 : Outport
  wires:
  Mux2/1 -> IEEE1547a_Volt/1
  Constant3/1 -> Mux1/1, Mux2/1
  Constant1/1 -> Mux1/2, Mux2/2
  Bus to Vector5/1 -> Mux2/3
  Bus Selector5/1 -> Bus to Vector5/1
  [F3_RELAY_OUT] -> Bus Selector5/1
  Mux1/1 -> IEEE1547a_Hz/1
  Bus to Vector1/1 -> Mux1/3
  Bus Selector1/1 -> Bus to Vector1/1
  [F3_RELAY_OUT] -> Bus Selector1/1
  Bus to Vector3/1 -> Mux2/4
  Bus Selector2/1 -> Bus to Vector3/1
  [F4_RELAY_OUT] -> Bus Selector7/1
  [F4_RELAY_OUT] -> Bus Selector2/1
  Bus to Vector/1 -> Mux1/4
  IEEE1547a_Hz/1 -> Mux3/1
  IEEE1547a_Volt/1 -> Mux3/2
  Mux3/1 -> Out1/1
  Bus Selector7/1 -> Bus to Vector/1
  Rst/1 -> IEEE1547a_Hz/2, IEEE1547a_Volt/2

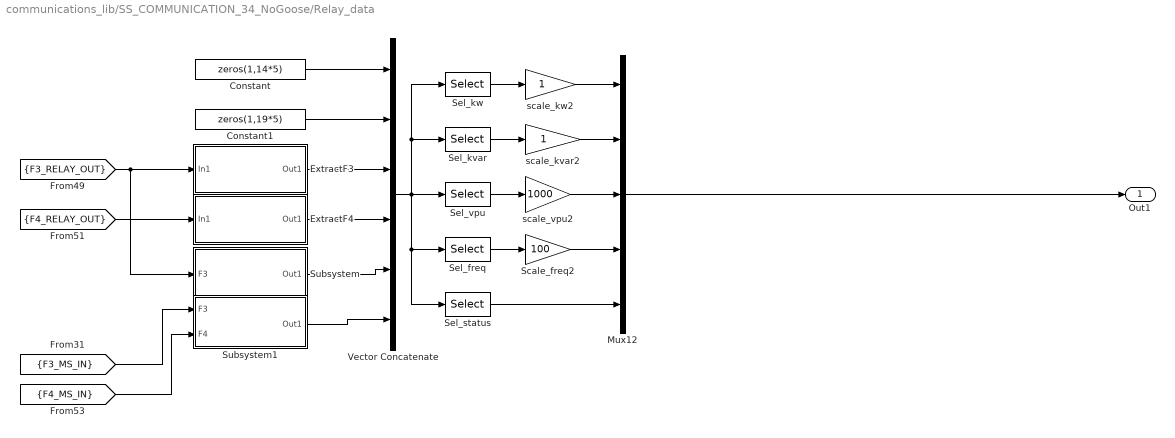
== system communications_lib/SS_COMMUNICATION_34_NoGoose/Relay_data ==
  Constant : Constant  Value=zeros(1,14*5)
  Constant1 : Constant  Value=zeros(1,19*5)
  ExtractF3 : Subsystem
      mask Display: disp('Generic F3 relays\nID = 34 .. 43')
  ExtractF4 : Subsystem
      mask Display: disp('Generic F4 relays\nID = 44 .. 49')
  Mux12 : Mux  Inputs=5
  Scale_freq2 : Gain  Gain=100
  Sel_freq : Selector  InputPortWidth=59*5  IndexOptions=Index vector (dialog)  Indices=[4:5:59*5]  OutputSizes=1
  Sel_kvar : Selector  InputPortWidth=59*5  IndexOptions=Index vector (dialog)  Indices=[2:5:59*5]  OutputSizes=1
  Sel_kw : Selector  InputPortWidth=59*5  IndexOptions=Index vector (dialog)  Indices=[1:5:59*5]  OutputSizes=1
  Sel_status : Selector  InputPortWidth=59*5  IndexOptions=Index vector (dialog)  Indices=[5:5:59*5]  OutputSizes=1
  Sel_vpu : Selector  InputPortWidth=59*5  IndexOptions=Index vector (dialog)  Indices=[3:5:59*5]  OutputSizes=1
  Subsystem : Subsystem
      mask Display: disp('Generic PCC relays\nID = 50 .. 52')
  Subsystem1 : Subsystem
      mask Display: disp('GEN1,ESS1,PV1\nGEN2,GEN3,ESS2,PV1\nID = 53 .. 59')
  Vector Concatenate : Concatenate  NumInputs=6
  scale_kvar2 : Gain
  scale_kw2 : Gain
  scale_vpu2 : Gain  Gain=1000
  Out1 : Outport
  wires:
  Vector Concatenate/1 -> Sel_kw/1, Sel_kvar/1, Sel_vpu/1, Sel_freq/1, Sel_status/1
  Sel_kvar/1 -> scale_kvar2/1
  Sel_vpu/1 -> scale_vpu2/1
  Sel_freq/1 -> Scale_freq2/1
  Sel_status/1 -> Mux12/5
  Sel_kw/1 -> scale_kw2/1
  scale_vpu2/1 -> Mux12/3
  Scale_freq2/1 -> Mux12/4
  scale_kvar2/1 -> Mux12/2
  scale_kw2/1 -> Mux12/1
  Mux12/1 -> Out1/1
  Subsystem1/1(Out1) -> Vector Concatenate/6
  [F3_MS_IN] -> Subsystem1/1(F3)
  [F4_MS_IN] -> Subsystem1/2(F4)
  Subsystem/1(Out1) -> Vector Concatenate/5
  Constant/1 -> Vector Concatenate/1
  Constant1/1 -> Vector Concatenate/2
  ExtractF3/1(Out1) -> Vector Concatenate/3
  ExtractF4/1(Out1) -> Vector Concatenate/4
  [F4_RELAY_OUT] -> ExtractF4/1(In1)
  [F3_RELAY_OUT] -> ExtractF3/1(In1), Subsystem/1(F3)

== system communications_lib/SS_COMMUNICATION_34_NoGoose/Time_ms ==
  Constant4 : Constant  Value=Ts/1e-3
  Sum : Sum  Inputs=++|
  Unit Delay : UnitDelay  SampleTime=-1
  Simtime_ms : Outport
  wires:
  Sum/1 -> Simtime_ms/1, Unit Delay/1
  Constant4/1 -> Sum/2
  Unit Delay/1 -> Sum/1

== system communications_lib/SS_COMMUNICATION/MGC_controller/Subsystem ==
  Bus Selector18 : BusSelector  OutputSignals=F3_CB_CTRL
  Bus Selector19 : BusSelector  OutputSignals=signal11
  Bus Selector20 : BusSelector  OutputSignals=F2_CB_CTRL
  Bus Selector21 : BusSelector  OutputSignals=signal20
  Bus Selector22 : BusSelector  OutputSignals=F1_CB_CTRL
  Bus Selector23 : BusSelector  OutputSignals=signal15
  Mux : Mux  Inputs=3
  Out1 : Outport
  wires:
  [F2_RELAY_OUT] -> Bus Selector20/1
  Bus Selector23/1 -> Mux/1  "<signal15>"
  [F3_RELAY_OUT] -> Bus Selector18/1
  [F1_RELAY_OUT] -> Bus Selector22/1
  Bus Selector22/1 -> Bus Selector23/1  "<F1_CB_CTRL>"
  Bus Selector21/1 -> Mux/2  "<signal20>"
  Mux/1 -> Out1/1
  Bus Selector18/1 -> Bus Selector19/1  "<F3_CB_CTRL>"
  Bus Selector19/1 -> Mux/3  "<signal11>"
  Bus Selector20/1 -> Bus Selector21/1  "<F2_CB_CTRL>"

== system communications_lib/SS_COMMUNICATION/Misc_data/Subsystem ==
  In1 : Inport
  Bus Selector28 : BusSelector  OutputSignals=F1.LOAD_DATA.F1_I1.kw,F1.LOAD_DATA.F1_I2.kw,F2.LOAD_DATA.F2_I3.kw,F2.LOAD_DATA.F2_I4.kw,F2.LOAD_DATA.F2_I5.kw,F3.LOAD_DATA.F3_I6.kw,F4.LOAD_DATA.F4_I7.kw,F4.LOAD_DATA.F4_I8.kw,F1.LOAD_DATA.F1_P1.kw,F2.LOAD_DATA.F2_P2.kw,F2.LOAD_DATA.F2_P3.kw,F3.LOAD_DATA.F3_P4.kw,F2.LOAD_DATA.F2_P5.kw,F3.LOAD_DATA.F3_P6.kw,F4.LOAD_DATA.F4_P7.kw,F4.LOAD_DATA.F4_P8.kw,F1.LOAD_DATA.F1_C1.kw,F1.LOAD_DATA.F1_C2.kw,F2.LOAD_DATA.F2_C3.kw,F2.LOAD_DATA.F2_C4.kw,F3.LOAD_DATA.F3_C5.kw,F3.LOAD_DATA.F3_C6.kw,F4.LOAD_DATA.F4_C7.kw,F4.LOAD_DATA.F4_C8.kw,F4.LOAD_DATA.F4_C9.kw
  Mux : Mux  Inputs=25
  Out1 : Outport
  wires:
  Mux/1 -> Out1/1
  Bus Selector28/14 -> Mux/14  "<kw>"
  Bus Selector28/5 -> Mux/5  "<kw>"
  Bus Selector28/15 -> Mux/15  "<kw>"
  Bus Selector28/8 -> Mux/8  "<kw>"
  Bus Selector28/6 -> Mux/6  "<kw>"
  Bus Selector28/16 -> Mux/16  "<kw>"
  Bus Selector28/17 -> Mux/17  "<kw>"
  Bus Selector28/4 -> Mux/4  "<kw>"
  Bus Selector28/25 -> Mux/25  "<kw>"
  Bus Selector28/23 -> Mux/23  "<kw>"
  Bus Selector28/24 -> Mux/24  "<kw>"
  Bus Selector28/22 -> Mux/22  "<kw>"
  Bus Selector28/13 -> Mux/13  "<kw>"
  Bus Selector28/2 -> Mux/2  "<kw>"
  Bus Selector28/7 -> Mux/7  "<kw>"
  Bus Selector28/11 -> Mux/11  "<kw>"
  Bus Selector28/20 -> Mux/20  "<kw>"
  Bus Selector28/10 -> Mux/10  "<kw>"
  Bus Selector28/18 -> Mux/18  "<kw>"
  Bus Selector28/21 -> Mux/21  "<kw>"
  Bus Selector28/12 -> Mux/12  "<kw>"
  Bus Selector28/9 -> Mux/9  "<kw>"
  Bus Selector28/3 -> Mux/3  "<kw>"
  Bus Selector28/19 -> Mux/19  "<kw>"
  Bus Selector28/1 -> Mux/1  "<kw>"
  In1/1 -> Bus Selector28/1

== system communications_lib/SS_COMMUNICATION/Misc_data/Subsystem1 ==
  In1 : Inport
  Bus Selector29 : BusSelector  OutputSignals=F1.LOAD_DATA.F1_I1.VRMSLL,F1.LOAD_DATA.F1_I2.VRMSLL,F2.LOAD_DATA.F2_I3.VRMSLL,F2.LOAD_DATA.F2_I4.VRMSLL,F2.LOAD_DATA.F2_I5.VRMSLL,F3.LOAD_DATA.F3_I6.VRMSLL,F4.LOAD_DATA.F4_I7.VRMSLL,F4.LOAD_DATA.F4_I8.VRMSLL,F1.LOAD_DATA.F1_P1.VRMSLL,F2.LOAD_DATA.F2_P2.VRMSLL,F2.LOAD_DATA.F2_P3.VRMSLL,F3.LOAD_DATA.F3_P4.VRMSLL,F2.LOAD_DATA.F2_P5.VRMSLL,F3.LOAD_DATA.F3_P6.VRMSLL,F4.LOAD_DATA.F4_P7.VRMSLL,F4.LOAD_DATA.F4_P8.VRMSLL,F1.LOAD_DATA.F1_C1.VRMSLL,F1.LOAD_DATA.F1_C2.VRMSLL,F2.LOAD_DATA.F2_C3.VRMSLL,F2.LOAD_DATA.F2_C4.VRMSLL,F3.LOAD_DATA.F3_C5.VRMSLL,F3.LOAD_DATA.F3_C6.VRMSLL,F4.LOAD_DATA.F4_C7.VRMSLL,F4.LOAD_DATA.F4_C8.VRMSLL,F4.LOAD_DATA.F4_C9.VRMSLL
  Mux : Mux  Inputs=25
  Out1 : Outport
  wires:
  Bus Selector29/13 -> Mux/13  "<VRMSLL>"
  Bus Selector29/14 -> Mux/14  "<VRMSLL>"
  Bus Selector29/15 -> Mux/15  "<VRMSLL>"
  Bus Selector29/16 -> Mux/16  "<VRMSLL>"
  Bus Selector29/17 -> Mux/17  "<VRMSLL>"
  Bus Selector29/18 -> Mux/18  "<VRMSLL>"
  Bus Selector29/19 -> Mux/19  "<VRMSLL>"
  Bus Selector29/20 -> Mux/20  "<VRMSLL>"
  Bus Selector29/21 -> Mux/21  "<VRMSLL>"
  Bus Selector29/22 -> Mux/22  "<VRMSLL>"
  Bus Selector29/23 -> Mux/23  "<VRMSLL>"
  Bus Selector29/24 -> Mux/24  "<VRMSLL>"
  Bus Selector29/25 -> Mux/25  "<VRMSLL>"
  Bus Selector29/3 -> Mux/3  "<VRMSLL>"
  Bus Selector29/4 -> Mux/4  "<VRMSLL>"
  Bus Selector29/2 -> Mux/2  "<VRMSLL>"
  Bus Selector29/6 -> Mux/6  "<VRMSLL>"
  Bus Selector29/5 -> Mux/5  "<VRMSLL>"
  Bus Selector29/8 -> Mux/8  "<VRMSLL>"
  Bus Selector29/7 -> Mux/7  "<VRMSLL>"
  Bus Selector29/10 -> Mux/10  "<VRMSLL>"
  Bus Selector29/9 -> Mux/9  "<VRMSLL>"
  Bus Selector29/12 -> Mux/12  "<VRMSLL>"
  Bus Selector29/11 -> Mux/11  "<VRMSLL>"
  Bus Selector29/1 -> Mux/1  "<VRMSLL>"
  In1/1 -> Bus Selector29/1
  Mux/1 -> Out1/1

== system communications_lib/SS_COMMUNICATION/Relay_data/ExtractF1 ==
  In1 : Inport
  Bus Selector47 : BusSelector  OutputSignals=F1_CB_1,F1_CB_2,F1_CB_3,F1_CB_4,F1_CB_5,F1_CB_6,F1_CB_7,F1_CB_8,F1_CB_9,F1_CB_10,F1_CB_11,F1_CB_12,F1_CB_13,F1_CB_14
  Bus Selector{48..53,56,58..64} (14 alike) : BusSelector  OutputSignals=m.kw,m.kvar,m.Vpu,m.Hz,m.status  OutputAsBus=on
  Mux13 : Mux  Inputs=14
  Out1 : Outport
  wires:
  Bus Selector63/1 -> Mux13/13
  Bus Selector61/1 -> Mux13/3
  Bus Selector62/1 -> Mux13/12
  Bus Selector59/1 -> Mux13/10
  Bus Selector47/5 -> Bus Selector51/1  "<F1_CB_5>"
  Bus Selector47/10 -> Bus Selector59/1  "<F1_CB_10>"
  Bus Selector49/1 -> Mux13/2
  Bus Selector47/14 -> Bus Selector64/1  "<F1_CB_14>"
  Bus Selector47/2 -> Bus Selector49/1  "<F1_CB_2>"
  Bus Selector47/3 -> Bus Selector61/1  "<F1_CB_3>"
  Bus Selector47/9 -> Bus Selector58/1  "<F1_CB_9>"
  Bus Selector47/8 -> Bus Selector56/1  "<F1_CB_8>"
  Bus Selector47/12 -> Bus Selector62/1  "<F1_CB_12>"
  Bus Selector47/7 -> Bus Selector53/1  "<F1_CB_7>"
  Bus Selector64/1 -> Mux13/14
  Bus Selector47/6 -> Bus Selector52/1  "<F1_CB_6>"
  Bus Selector58/1 -> Mux13/9
  Bus Selector56/1 -> Mux13/8
  Bus Selector52/1 -> Mux13/6
  Bus Selector47/11 -> Bus Selector60/1  "<F1_CB_11>"
  Bus Selector60/1 -> Mux13/11
  Mux13/1 -> Out1/1
  In1/1 -> Bus Selector47/1
  Bus Selector50/1 -> Mux13/4
  Bus Selector47/1 -> Bus Selector48/1  "<F1_CB_1>"
  Bus Selector47/4 -> Bus Selector50/1  "<F1_CB_4>"
  Bus Selector53/1 -> Mux13/7
  Bus Selector48/1 -> Mux13/1
  Bus Selector51/1 -> Mux13/5
  Bus Selector47/13 -> Bus Selector63/1  "<F1_CB_13>"

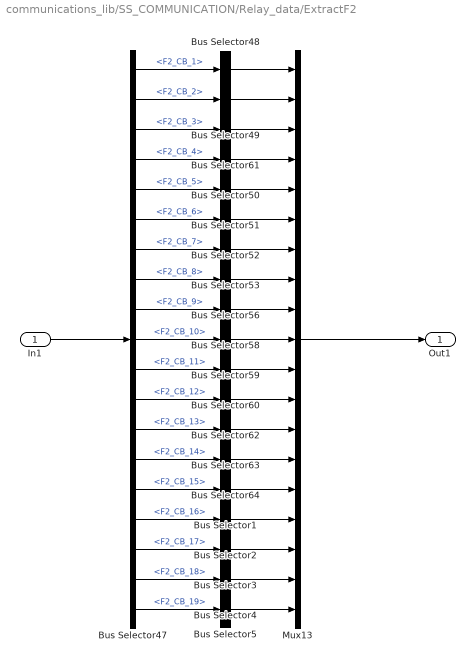
== system communications_lib/SS_COMMUNICATION/Relay_data/ExtractF2 ==
  In1 : Inport
  Bus Selector{1..5,48..53,56,58..64} (19 alike) : BusSelector  OutputSignals=m.kw,m.kvar,m.Vpu,m.Hz,m.status  OutputAsBus=on
  Bus Selector47 : BusSelector  OutputSignals=F2_CB_1,F2_CB_2,F2_CB_3,F2_CB_4,F2_CB_5,F2_CB_6,F2_CB_7,F2_CB_8,F2_CB_9,F2_CB_10,F2_CB_11,F2_CB_12,F2_CB_13,F2_CB_14,F2_CB_15,F2_CB_16,F2_CB_17,F2_CB_18,F2_CB_19
  Mux13 : Mux  Inputs=19
  Out1 : Outport
  wires:
  Bus Selector47/18 -> Bus Selector4/1  "<F2_CB_18>"
  Bus Selector2/1 -> Mux13/16
  Bus Selector47/16 -> Bus Selector2/1  "<F2_CB_16>"
  Bus Selector5/1 -> Mux13/19
  Bus Selector47/17 -> Bus Selector3/1  "<F2_CB_17>"
  Bus Selector47/19 -> Bus Selector5/1  "<F2_CB_19>"
  Bus Selector47/15 -> Bus Selector1/1  "<F2_CB_15>"
  Bus Selector1/1 -> Mux13/15
  Bus Selector3/1 -> Mux13/17
  Bus Selector4/1 -> Mux13/18
  Bus Selector47/13 -> Bus Selector63/1  "<F2_CB_13>"
  Bus Selector51/1 -> Mux13/5
  Bus Selector48/1 -> Mux13/1
  Bus Selector53/1 -> Mux13/7
  Bus Selector47/4 -> Bus Selector50/1  "<F2_CB_4>"
  Bus Selector47/1 -> Bus Selector48/1  "<F2_CB_1>"
  Bus Selector50/1 -> Mux13/4
  In1/1 -> Bus Selector47/1
  Mux13/1 -> Out1/1
  Bus Selector60/1 -> Mux13/11
  Bus Selector47/11 -> Bus Selector60/1  "<F2_CB_11>"
  Bus Selector52/1 -> Mux13/6
  Bus Selector56/1 -> Mux13/8
  Bus Selector58/1 -> Mux13/9
  Bus Selector47/6 -> Bus Selector52/1  "<F2_CB_6>"
  Bus Selector64/1 -> Mux13/14
  Bus Selector47/7 -> Bus Selector53/1  "<F2_CB_7>"
  Bus Selector47/12 -> Bus Selector62/1  "<F2_CB_12>"
  Bus Selector47/8 -> Bus Selector56/1  "<F2_CB_8>"
  Bus Selector47/9 -> Bus Selector58/1  "<F2_CB_9>"
  Bus Selector47/3 -> Bus Selector61/1  "<F2_CB_3>"
  Bus Selector47/2 -> Bus Selector49/1  "<F2_CB_2>"
  Bus Selector47/14 -> Bus Selector64/1  "<F2_CB_14>"
  Bus Selector49/1 -> Mux13/2
  Bus Selector47/10 -> Bus Selector59/1  "<F2_CB_10>"
  Bus Selector47/5 -> Bus Selector51/1  "<F2_CB_5>"
  Bus Selector59/1 -> Mux13/10
  Bus Selector62/1 -> Mux13/12
  Bus Selector61/1 -> Mux13/3
  Bus Selector63/1 -> Mux13/13

== system communications_lib/SS_COMMUNICATION/Relay_data/ExtractF3 ==
  In1 : Inport
  Bus Selector47 : BusSelector  OutputSignals=F3_CB_1,F3_CB_2,F3_CB_3,F3_CB_4,F3_CB_5,F3_CB_6,F3_CB_7,F3_CB_8,F3_CB_9,F3_CB_10
  Bus Selector{48..53,56,58..59,61} (10 alike) : BusSelector  OutputSignals=m.kw,m.kvar,m.Vpu,m.Hz,m.status  OutputAsBus=on
  Mux13 : Mux  Inputs=10
  Out1 : Outport
  wires:
  Bus Selector61/1 -> Mux13/3
  Bus Selector59/1 -> Mux13/10
  Bus Selector47/5 -> Bus Selector51/1  "<F3_CB_5>"
  Bus Selector47/10 -> Bus Selector59/1  "<F3_CB_10>"
  Bus Selector49/1 -> Mux13/2
  Bus Selector47/2 -> Bus Selector49/1  "<F3_CB_2>"
  Bus Selector47/3 -> Bus Selector61/1  "<F3_CB_3>"
  Bus Selector47/9 -> Bus Selector58/1  "<F3_CB_9>"
  Bus Selector47/8 -> Bus Selector56/1  "<F3_CB_8>"
  Bus Selector47/7 -> Bus Selector53/1  "<F3_CB_7>"
  Bus Selector47/6 -> Bus Selector52/1  "<F3_CB_6>"
  Bus Selector58/1 -> Mux13/9
  Bus Selector56/1 -> Mux13/8
  Bus Selector52/1 -> Mux13/6
  Mux13/1 -> Out1/1
  In1/1 -> Bus Selector47/1
  Bus Selector50/1 -> Mux13/4
  Bus Selector47/1 -> Bus Selector48/1  "<F3_CB_1>"
  Bus Selector47/4 -> Bus Selector50/1  "<F3_CB_4>"
  Bus Selector53/1 -> Mux13/7
  Bus Selector48/1 -> Mux13/1
  Bus Selector51/1 -> Mux13/5

== system communications_lib/SS_COMMUNICATION/Relay_data/ExtractF4 ==
  In1 : Inport
  Bus Selector47 : BusSelector  OutputSignals=F4_CB_1,F4_CB_2,F4_CB_3,F4_CB_4,F4_CB_5,F4_CB_6
  Bus Selector{48..52,61} (6 alike) : BusSelector  OutputSignals=m.kw,m.kvar,m.Vpu,m.Hz,m.status  OutputAsBus=on
  Mux13 : Mux  Inputs=6
  Out1 : Outport
  wires:
  Bus Selector51/1 -> Mux13/5
  Bus Selector48/1 -> Mux13/1
  Bus Selector47/4 -> Bus Selector50/1  "<F4_CB_4>"
  Bus Selector47/1 -> Bus Selector48/1  "<F4_CB_1>"
  Bus Selector50/1 -> Mux13/4
  In1/1 -> Bus Selector47/1
  Mux13/1 -> Out1/1
  Bus Selector52/1 -> Mux13/6
  Bus Selector47/6 -> Bus Selector52/1  "<F4_CB_6>"
  Bus Selector47/3 -> Bus Selector61/1  "<F4_CB_3>"
  Bus Selector47/2 -> Bus Selector49/1  "<F4_CB_2>"
  Bus Selector49/1 -> Mux13/2
  Bus Selector47/5 -> Bus Selector51/1  "<F4_CB_5>"
  Bus Selector61/1 -> Mux13/3

== system communications_lib/SS_COMMUNICATION/Relay_data/Subsystem ==
  F1 : Inport
  F2 : Inport  Port=2
  F3 : Inport  Port=3
  Bus Selector1 : BusSelector  OutputSignals=F2_PCC
  Bus Selector2 : BusSelector  OutputSignals=m.kw,m.kvar,m.Vpu,m.Hz,m.status  OutputAsBus=on
  Bus Selector3 : BusSelector  OutputSignals=F3_PCC
  Bus Selector4 : BusSelector  OutputSignals=m.kw,m.kvar,m.Vpu,m.Hz,m.status  OutputAsBus=on
  Bus Selector47 : BusSelector  OutputSignals=F1_PCC
  Bus Selector48 : BusSelector  OutputSignals=m.kw,m.kvar,m.Vpu,m.Hz,m.status  OutputAsBus=on
  Mux : Mux  Inputs=3
  Out1 : Outport
  wires:
  Mux/1 -> Out1/1
  Bus Selector4/1 -> Mux/3
  F3/1 -> Bus Selector3/1
  Bus Selector3/1 -> Bus Selector4/1  "<F3_PCC>"
  Bus Selector2/1 -> Mux/2
  F2/1 -> Bus Selector1/1
  Bus Selector1/1 -> Bus Selector2/1  "<F2_PCC>"
  Bus Selector48/1 -> Mux/1
  F1/1 -> Bus Selector47/1
  Bus Selector47/1 -> Bus Selector48/1  "<F1_PCC>"

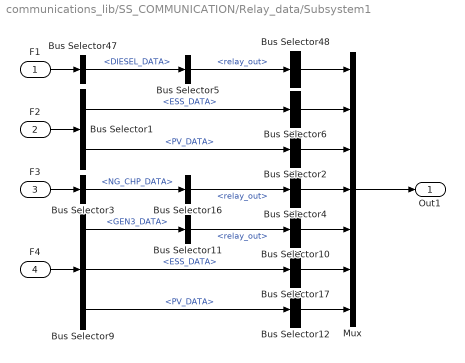
== system communications_lib/SS_COMMUNICATION/Relay_data/Subsystem1 ==
  F1 : Inport
  F2 : Inport  Port=2
  F3 : Inport  Port=3
  F4 : Inport  Port=4
  Bus Selector1 : BusSelector  OutputSignals=ESS_DATA,PV_DATA
  Bus Selector10 : BusSelector  OutputSignals=m.kw,m.kvar,m.Vpu,m.Hz,m.status  OutputAsBus=on
  Bus Selector11 : BusSelector  OutputSignals=cb.relay_out
  Bus Selector{2,6,12,17} (4 alike) : BusSelector  OutputSignals=CB_meas.relay_out.m.kw,CB_meas.relay_out.m.kvar,CB_meas.relay_out.m.Vpu,CB_meas.relay_out.m.Hz,CB_meas.cb_meas.Status  OutputAsBus=on
  Bus Selector16 : BusSelector  OutputSignals=cb.relay_out
  Bus Selector3 : BusSelector  OutputSignals=NG_CHP_DATA
  Bus Selector4 : BusSelector  OutputSignals=m.kw,m.kvar,m.Vpu,m.Hz,m.status  OutputAsBus=on
  Bus Selector47 : BusSelector  OutputSignals=DIESEL_DATA
  Bus Selector48 : BusSelector  OutputSignals=m.kw,m.kvar,m.Vpu,m.Hz,m.status  OutputAsBus=on
  Bus Selector5 : BusSelector  OutputSignals=cb.relay_out
  Bus Selector9 : BusSelector  OutputSignals=GEN3_DATA,ESS_DATA,PV_DATA
  Mux : Mux  Inputs=7
  Out1 : Outport
  wires:
  Bus Selector9/2 -> Bus Selector17/1  "<ESS_DATA>"
  Bus Selector16/1 -> Bus Selector4/1  "<relay_out>"
  Bus Selector12/1 -> Mux/7
  Bus Selector9/3 -> Bus Selector12/1  "<PV_DATA>"
  Bus Selector17/1 -> Mux/6
  Bus Selector10/1 -> Mux/5
  Bus Selector11/1 -> Bus Selector10/1  "<relay_out>"
  Bus Selector9/1 -> Bus Selector11/1  "<GEN3_DATA>"
  F4/1 -> Bus Selector9/1
  Bus Selector2/1 -> Mux/3
  Bus Selector1/2 -> Bus Selector2/1  "<PV_DATA>"
  Bus Selector5/1 -> Bus Selector48/1  "<relay_out>"
  Bus Selector47/1 -> Bus Selector5/1  "<DIESEL_DATA>"
  F1/1 -> Bus Selector47/1
  Bus Selector48/1 -> Mux/1
  Bus Selector1/1 -> Bus Selector6/1  "<ESS_DATA>"
  F2/1 -> Bus Selector1/1
  Bus Selector6/1 -> Mux/2
  Bus Selector3/1 -> Bus Selector16/1  "<NG_CHP_DATA>"
  F3/1 -> Bus Selector3/1
  Bus Selector4/1 -> Mux/4
  Mux/1 -> Out1/1
